simulink model "Assem2"  (R2015b)
settings: Solver=FixedStepAuto  StartTime=0.0  StopTime=10.0  RelTol=1e-3
undefined symbols (not defined in the file): pendulum, support
libraries: mblibv1 x9, arduinolib x2
settings Model: ExtModeTrigDuration=2  Creator=kedar  LastModifiedBy=kedar
settings OptimizationCC: OptimizeModelRefInitCode=on  LifeSpan=1  MaxStackSize=64
settings HardwareCC: ProdBitPerInt=16  ProdBitPerPointer=16  ProdLargestAtomicFloat=None  ProdWordSize=8  ProdHWDeviceType=Atmel->AVR
settings RTWCC: SystemTargetFile=ert.tlc  TemplateMakefile=ert_default_tmf  Description=Embedded Coder  Toolchain=Arduino AVR v1.6.1  BuildConfiguration=Faster Runs
settings CodeAppCC: IgnoreCustomStorageClasses=off
settings ERTTargetCC: GenerateSampleERTMain=on  SupportContinuousTime=on  SupportVariableSizeSignals=on
settings SimMechanicsCC: VisOnUpdateDiagram=on  VisDuringSimulation=on

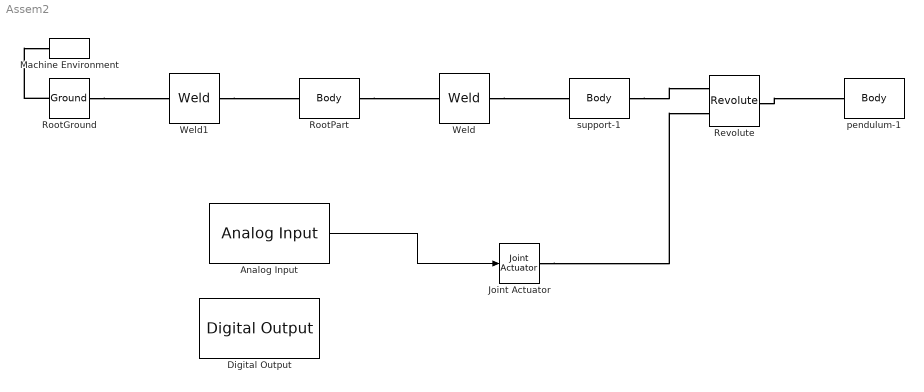
== system Assem2 ==
  Analog Input : arduinolib/Analog Input  pinNumber=4  sampleTime=1  blockPlatform=arduino
  Digital Output : arduinolib/Digital Output  pinNumber=9  blockPlatform=arduino
  Joint Actuator : mblibv1/Sensors &  Actuators/Joint Actuator  UpdateFromCAD=off  PhysicalDomain=Mechanical  PortType=blob  ActuationStyle=Force  AngleUnits=rev  ArcVelocityUnits=rpm  ArcAccelerationUnits=rad/s^2  CoordPositionUnits=m  VelocityUnits=m/s  AccelerationUnits=m/s^2  ForceUnits=N  TorqueUnits=N*m  ActiveIO=on  Width=1  DialogClass=MechanicalActuatorBlock  Primitive=R1  ReferenceFrame=Absolute (World)
  Machine Environment : mblibv1/Bodies/Machine Environment  PortType=env  PhysicalDomain=Mechanical  DialogTemplateClass=MECH.MachineEnvironment  SyncWhenCopied=off  Gravity=[0 -9.81 0]  GravityUnits=m/s^2  GravityAsSignal=off  Dimensionality=Auto-detect  AnalysisType=Forward dynamics  LinearAssemblyTolerance=1e-3  LinearAssemblyToleranceUnits=m  AngularAssemblyTolerance=1e-3  AngularAssemblyToleranceUnits=rad  ConstraintSolverType=Stabilizing  ConstraintRelTolerance=1e-4  ConstraintAbsTolerance=1e-4  UseRobustSingularityHandling=off  RedundancyAnalysisToleranceType=Automatically select tolerance  RedundancyAnalysisTolerance=1e-14  StatePerturbationType=Fixed  PerturbationSize=1e-5  VisualizeMachine=on  BodyVisualizationType=Use model default body geometries  BodyColorSelMode=Use model default  DefaultBodyColor=[1 0 0]
  Revolute : mblibv1/Joints/Revolute  LConnTagsString=__newl0|SA1  RConnTagsString=__newr0  UpdateFromCAD=on  PMImportedID=pendulum-1:-:support-1  NumSAPorts=1  CutJoint=off  MarkAsCut=off  Primitives=prismatic  PrimitiveProps=R1$World$[-1,0,0]$revolute  DialogClass=JointBlock  R1Axis=[-1,0,0]
  RootGround : mblibv1/Bodies/Ground  UpdateFromCAD=on  PMImportedID=RootGround  LeftPortType=env  RightPortType=workingframe  PhysicalDomain=Mechanical  DialogClass=GroundBlock  CoordPosition=[-0.00495247,-0.0191756,0.105201]  CoordPositionUnits=m  StateVectorMgrId=1  MachineId=[1 0]  ShowEnvPort=on  ParameterChecksum=[194244226, 1977581229, 4183864686, 3123721425]  TopologyChecksum=[3149135417, 452869324, 3965643881, 3197160252]
  RootPart : mblibv1/Bodies/Body  LConnTagsString=CS3  RConnTagsString=CS2  UpdateFromCAD=on  PMImportedID=Assem2/RootPart  DialogClass=MechanicalBodyBlock  Mass=0  MassUnits=kg  InertiaUnits=kg*m^2  Inertia=[0,0,0;0,0,0;0,0,0]  Shape=Cylinder  ShapeDims=[1 1]  ShapeUnits=m  ShapeUse=false  Density=1  DensityUnits=kg/m^3  DensityUse=false  GraphicsMode=MACHINE_DEFAULT  BodyColorSelMode=MACHINE_DEFAULT  BodyColor=[1;0;0]  AttachedToCS=CS1  CG=Right$CG$[-0.00495247 -0.0191756 0.105201]$WORLD$WORLD$m$[1 0 0;0 1 0;0 0 1]$3x3 Transform$rad$WORLD$false$Assem2/RootPart::CG(AUTOGEN)  WorkingFrames=Right$CS1$[0 0 0]$WORLD$WORLD$m$[1 0 0;0 1 0;0 0 1]$3x3 Transform$rad$WORLD$false$Assem2/RootPart::CS1(AUTOGEN)#Right$CS2$[0.00290946 0.0201907 0.0401498]$WORLD$WORLD$m$[1 0 0;0 1 0;0 0 1]$3x3 Transform$rad$WORLD$true$Assem2/RootPart:-:support-1::Assem2/RootPart(AUTOGEN)#Left$CS3$[-0.00495247 -0.0191756 0.105201]$WORLD$WORLD$m$[1 0 0;0 1 0;0 0 1]$3x3 Transform$rad$WORLD$true$Assem2/RootPart:-:RootGround::Assem2/RootPart(AUTOGEN)  CGPos=[-0.00495247 -0.0191756 0.105201]  CGRot=[1 0 0;0 1 0;0 0 1]  CS0Pos=[]  CS0Rot=[]  CS1Pos=[0 0 0]  CS1Rot=[1 0 0;0 1 0;0 0 1]  CS2Pos=[0.00290946 0.0201907 0.0401498]  CS2Rot=[1 0 0;0 1 0;0 0 1]  CS3Pos=[-0.00495247 -0.0191756 0.105201]  CS3Rot=[1 0 0;0 1 0;0 0 1]  CS4Pos=[]  CS4Rot=[]  CS5Pos=[]  CS5Rot=[]  CS6Pos=[]  CS6Rot=[]  CS7Pos=[]  CS7Rot=[]  CS8Pos=[]  CS8Rot=[]  CS9Pos=[]  CS9Rot=[]  CS10Pos=[]  CS10Rot=[]  CS11Pos=[]  CS11Rot=[]  CS12Pos=[]  CS12Rot=[]  CS13Pos=[]  CS13Rot=[]  CS14Pos=[]  CS14Rot=[]  CS15Pos=[]  CS15Rot=[]  CS16Pos=[]  CS16Rot=[]  CS17Pos=[]  CS17Rot=[]  CS18Pos=[]  CS18Rot=[]  CS19Pos=[]  CS19Rot=[]  CS20Pos=[]  CS20Rot=[]
  Weld : mblibv1/Joints/Weld  LConnTagsString=__newl0  RConnTagsString=__newr0  UpdateFromCAD=on  PMImportedID=Assem2/RootPart:-:support-1  NumSAPorts=0  CutJoint=off  MarkAsCut=off  Primitives=weld  PrimitiveProps=W$WORLD$[0.57735,0.57735,0.57735]$weld  DialogClass=JointBlock  WAxis=[0.57735,0.57735,0.57735]
  Weld1 : mblibv1/Joints/Weld  LConnTagsString=__newl0  RConnTagsString=__newr0  UpdateFromCAD=on  PMImportedID=Assem2/RootPart:-:RootGround  NumSAPorts=0  CutJoint=off  MarkAsCut=off  Primitives=weld  PrimitiveProps=W$WORLD$[0.57735,0.57735,0.57735]$weld  DialogClass=JointBlock  WAxis=[0.57735,0.57735,0.57735]
  pendulum-1 : mblibv1/Bodies/Body  LConnTagsString=CS2  UpdateFromCAD=on  PMImportedID=pendulum-1  DialogClass=MechanicalBodyBlock  Mass=0.0462081  MassUnits=kg  InertiaUnits=kg*m^2  Inertia=[5.07082e-06,-2.59516e-06,0;-2.59516e-06,0.000273575,0;0,0,0.000277875]  Shape=Cylinder  ShapeDims=[1 1]  ShapeUnits=m  ShapeUse=false  Density=1  DensityUnits=kg/m^3  DensityUse=false  GraphicsMode=GFXFILE  GraphicsFileName=Assem2 - pendulum-1.STL  BodyColorSelMode=COLORPALETTE  BodyColor=[0.79216 0.81961 0.93333]  AttachedToCS=CS1  CG=Right$CG$[-0.00709054 -0.0298813 0.122892]$WORLD$WORLD$m$[0 0 -1;-0.536318 0.844016 0;0.844016 0.536318 0]$3x3 Transform$rad$WORLD$false$pendulum-1::CG(AUTOGEN)  WorkingFrames=Right$CS1$[-0.00209054 0.0201907 0.0401498]$WORLD$WORLD$m$[0 0 -1;-0.536318 0.844016 0;0.844016 0.536318 0]$3x3 Transform$rad$WORLD$false$pendulum-1::CS1(AUTOGEN)#Left$CS2$[-0.00209054 0.0201907 0.0401498]$WORLD$WORLD$m$[1 0 0;0 1 0;0 0 1]$3x3 Transform$rad$WORLD$true$pendulum-1:-:support-1::pendulum-1(AUTOGEN)  CGPos=[-0.00709054 -0.0298813 0.122892]  CGRot=[0 0 -1;-0.536318 0.844016 0;0.844016 0.536318 0]  CS0Pos=[]  CS0Rot=[]  CS1Pos=[-0.00209054 0.0201907 0.0401498]  CS1Rot=[0 0 -1;-0.536318 0.844016 0;0.844016 0.536318 0]  CS2Pos=[-0.00209054 0.0201907 0.0401498]  CS2Rot=[1 0 0;0 1 0;0 0 1]  CS3Pos=[]  CS3Rot=[]  CS4Pos=[]  CS4Rot=[]  CS5Pos=[]  CS5Rot=[]  CS6Pos=[]  CS6Rot=[]  CS7Pos=[]  CS7Rot=[]  CS8Pos=[]  CS8Rot=[]  CS9Pos=[]  CS9Rot=[]  CS10Pos=[]  CS10Rot=[]  CS11Pos=[]  CS11Rot=[]  CS12Pos=[]  CS12Rot=[]  CS13Pos=[]  CS13Rot=[]  CS14Pos=[]  CS14Rot=[]  CS15Pos=[]  CS15Rot=[]  CS16Pos=[]  CS16Rot=[]  CS17Pos=[]  CS17Rot=[]  CS18Pos=[]  CS18Rot=[]  CS19Pos=[]  CS19Rot=[]  CS20Pos=[]  CS20Rot=[]
  support-1 : mblibv1/Bodies/Body  LConnTagsString=CS2  RConnTagsString=CS3  UpdateFromCAD=on  PMImportedID=support-1  DialogClass=MechanicalBodyBlock  Mass=0.0125664  MassUnits=kg  InertiaUnits=kg*m^2  Inertia=[2.51327e-06,0,0;0,1.36136e-06,0;0,0,1.36136e-06]  Shape=Cylinder  ShapeDims=[1 1]  ShapeUnits=m  ShapeUse=false  Density=1  DensityUnits=kg/m^3  DensityUse=false  GraphicsMode=GFXFILE  GraphicsFileName=Assem2 - support-1.STL  BodyColorSelMode=COLORPALETTE  BodyColor=[0.792157;0.819608;0.933333]  AttachedToCS=CS1  CG=Right$CG$[0.00290946 0.0201907 0.0401498]$WORLD$WORLD$m$[1 0 0;0 1 0;0 0 1]$3x3 Transform$rad$WORLD$false$support-1::CG(AUTOGEN)  WorkingFrames=Right$CS1$[-0.00209054 0.0201907 0.0401498]$WORLD$WORLD$m$[1 0 0;0 1 0;0 0 1]$3x3 Transform$rad$WORLD$false$support-1::CS1(AUTOGEN)#Left$CS2$[0.00290946 0.0201907 0.0401498]$WORLD$WORLD$m$[1 0 0;0 1 0;0 0 1]$3x3 Transform$rad$WORLD$true$Assem2/RootPart:-:support-1::support-1(AUTOGEN)#Right$CS3$[-0.00209054 0.0201907 0.0401498]$WORLD$WORLD$m$[1 0 0;0 1 0;0 0 1]$3x3 Transform$rad$WORLD$true$pendulum-1:-:support-1::support-1(AUTOGEN)  CGPos=[0.00290946 0.0201907 0.0401498]  CGRot=[1 0 0;0 1 0;0 0 1]  CS0Pos=[]  CS0Rot=[]  CS1Pos=[-0.00209054 0.0201907 0.0401498]  CS1Rot=[1 0 0;0 1 0;0 0 1]  CS2Pos=[0.00290946 0.0201907 0.0401498]  CS2Rot=[1 0 0;0 1 0;0 0 1]  CS3Pos=[-0.00209054 0.0201907 0.0401498]  CS3Rot=[1 0 0;0 1 0;0 0 1]  CS4Pos=[]  CS4Rot=[]  CS5Pos=[]  CS5Rot=[]  CS6Pos=[]  CS6Rot=[]  CS7Pos=[]  CS7Rot=[]  CS8Pos=[]  CS8Rot=[]  CS9Pos=[]  CS9Rot=[]  CS10Pos=[]  CS10Rot=[]  CS11Pos=[]  CS11Rot=[]  CS12Pos=[]  CS12Rot=[]  CS13Pos=[]  CS13Rot=[]  CS14Pos=[]  CS14Rot=[]  CS15Pos=[]  CS15Rot=[]  CS16Pos=[]  CS16Rot=[]  CS17Pos=[]  CS17Rot=[]  CS18Pos=[]  CS18Rot=[]  CS19Pos=[]  CS19Rot=[]  CS20Pos=[]  CS20Rot=[]
  wires:
  Analog Input/1 -> Joint Actuator/1
  connections:
  RootPart/RConn1 -- Weld/LConn1
  Weld/RConn1 -- support-1/LConn1
  Revolute/RConn1 -- pendulum-1/LConn1
  RootGround/RConn1 -- Weld1/LConn1
  Weld1/RConn1 -- RootPart/LConn1
  RootGround/LConn1 -- Machine Environment/RConn1
  support-1/RConn1 -- Revolute/LConn1
  Joint Actuator/RConn1 -- Revolute/LConn2
